simulink model "ex3_sim1"  (R2019b)
settings: Solver=ode45  StartTime=0.0  StopTime=2  MaxStep=0.001  RelTol=1e-3
undefined symbols (not defined in the file): Ad, Ar, denC1, denC2, denH, denP, kff, numC1, numC2, numH, numP, rads2rpm, t0d, t0r, Ts
Description:
  | Riccardo Antonello (riccardo.antonello@unipd.it)
  | 
  | June 18, 2020
  | 
  | Dept. of Information Engineering, University of Padova
settings Model: Creator=riccardo  LastModifiedBy=riccardo
settings DataIOCC: ReturnWorkspaceOutputs=off
settings DebuggingCC: ArithmeticOperatorsInVariantConditions=warning
settings SFSimCC: CustomCodeUndefinedFunction=UseInterfaceOnly

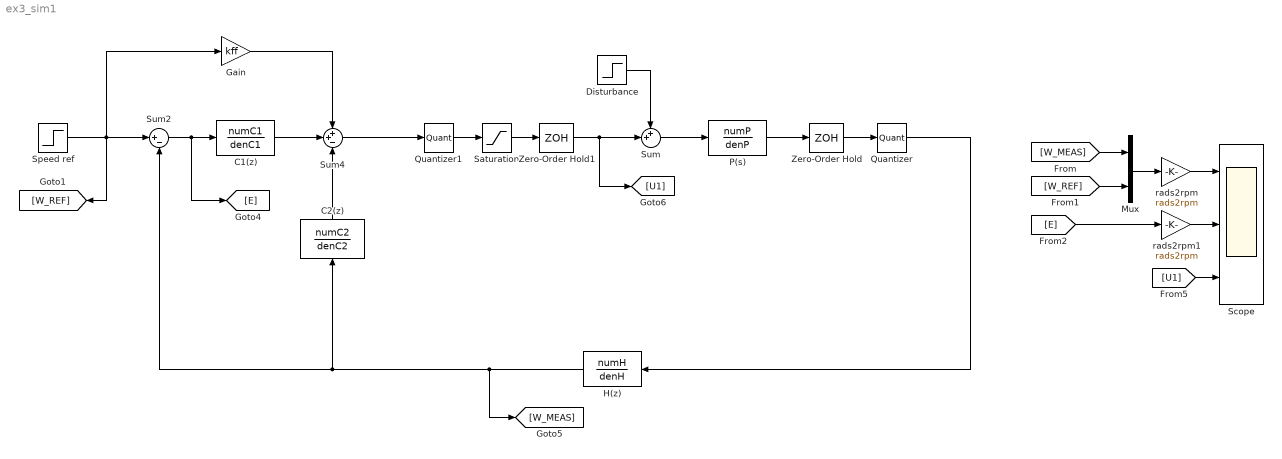
== system ex3_sim1 ==
  C1(z) : DiscreteTransferFcn  Numerator=numC1  Denominator=denC1  SampleTime=Ts
  C2(z) : DiscreteTransferFcn  Numerator=numC2  Denominator=denC2  SampleTime=Ts
  Disturbance : Step  Time=t0d  After=Ad  SampleTime=0
  Gain : Gain  Gain=kff
  H(z) : DiscreteTransferFcn  Numerator=numH  Denominator=denH  SampleTime=Ts
  Mux : Mux  Inputs=2
  P(s) : TransferFcn  Numerator=numP  Denominator=denP
  Quantizer : Quantizer  QuantizationInterval=2*pi/2000
  Quantizer1 : Quantizer  QuantizationInterval=20/2^10
  Saturation : Saturate  UpperLimit=10  LowerLimit=-10
  Scope : Scope  NumInputPorts=3
  Speed ref : Step  Time=t0r  After=Ar  SampleTime=Ts
  Sum : Sum  Inputs=++|
  Sum2 : Sum  Inputs=|+-
  Sum4 : Sum  Inputs=++-
  Zero-Order Hold : ZeroOrderHold  SampleTime=Ts
  Zero-Order Hold1 : ZeroOrderHold  SampleTime=Ts
  rads2rpm : Gain  Gain=rads2rpm
  rads2rpm1 : Gain  Gain=rads2rpm
  wires:
  Saturation/1 -> Zero-Order Hold1/1
  Sum2/1 -> [E], C1(z)/1
  Speed ref/1 -> Gain/1, Sum2/1, [W_REF]
  Sum4/1 -> Quantizer1/1
  Mux/1 -> rads2rpm/1
  [W_MEAS] -> Mux/1
  [W_REF] -> Mux/2
  [E] -> rads2rpm1/1
  rads2rpm/1 -> Scope/1
  Disturbance/1 -> Sum/1
  Zero-Order Hold/1 -> Quantizer/1
  Quantizer/1 -> H(z)/1
  Zero-Order Hold1/1 -> [U1], Sum/2
  Quantizer1/1 -> Saturation/1
  rads2rpm1/1 -> Scope/2
  P(s)/1 -> Zero-Order Hold/1
  [U1] -> Scope/3
  H(z)/1 -> [W_MEAS], C2(z)/1, Sum2/2
  Sum/1 -> P(s)/1
  C1(z)/1 -> Sum4/2
  C2(z)/1 -> Sum4/3
  Gain/1 -> Sum4/1
